simulink model "pController"  (R2024a)
settings: Solver=VariableStepAuto  StartTime=0.0  StopTime=0.1  FixedStep=1000  MaxStep=0.0001  RelTol=1e-3
values from neighbouring files (symbols this model uses):
  KR = KR_LIST(i)    [plotPController.m]
settings Model: Creator=janho  LastModifiedBy=janho

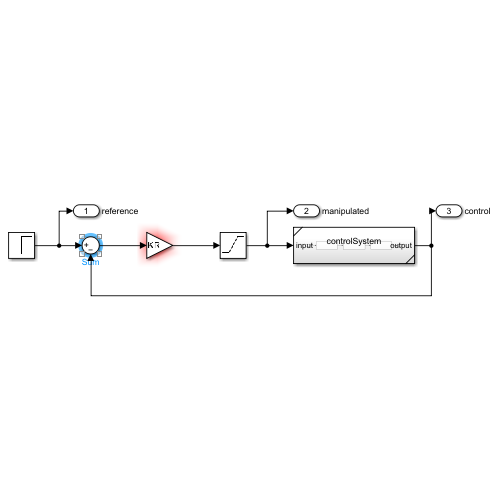
[thumbnail: Simulink's stored preview of the top-level diagram]
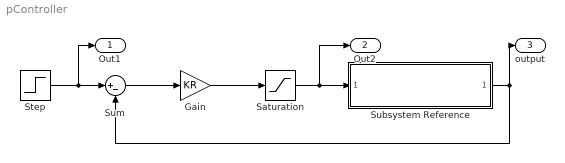
== system pController ==
  Gain : Gain  Gain=KR
  Saturation : Saturate  UpperLimit=12  LowerLimit=-12
  Step : Step  Time=0  After=4  SampleTime=0
  Subsystem Reference : Subsystem  ReferencedSubsystem=controlSystem
  Sum : Sum  Inputs=|+-
  Out1 : Outport  SignalName=reference
  Out2 : Outport  Port=2  SignalName=manipulated
  output : Outport  Port=3  SignalName=control
  wires:
  Step/1 -> Out1/1, Sum/1
  Sum/1 -> Gain/1
  Subsystem Reference/1 -> output/1, Sum/2
  Gain/1 -> Saturation/1
  Saturation/1 -> Out2/1, Subsystem Reference/1
